simulink model "ES247A_MotAgCmp"  (R2013b)
settings: Solver=VariableStepDiscrete  SolverMode=SingleTasking  StartTime=0.0  StopTime=1  FixedStep=0.002  RelTol=1e-3
values from neighbouring files (symbols this model uses):
  MOTAGCMPENAMASK_CNT_U08 = DataDict.Constant    [ES247A_MotAgCmp_DataDict.m]
  MOTAGCMPMECLDEGPERREV_DEGPERREV_U16P0 = DataDict.Constant    [ES247A_MotAgCmp_DataDict.m]
  MOTAGCUMVALGNDMASK_CNT_U32 = DataDict.Constant    [ES247A_MotAgCmp_DataDict.m]
  MOTAGCUMVALGNDMRFREVMASK_CNT_U32 = DataDict.Constant    [ES247A_MotAgCmp_DataDict.m]
  MOTAGDELTALIM_MOTREV_U0P16 = DataDict.Constant    [ES247A_MotAgCmp_DataDict.m]
  MOTAGMAXDELTA_MOTREV_U0P16 = DataDict.Constant    [ES247A_MotAgCmp_DataDict.m]
  SysGlbPrmMotPoleCnt = DataDict.ImprtdCal    [ES247A_MotAgCmp_DataDict.m]
  SysGlbPrmSysKineRat = DataDict.ImprtdCal    [ES247A_MotAgCmp_DataDict.m]
undefined symbols (not defined in the file or in its folder): sigbuilder_block
libraries: simulink x8, NexteerUtilities x4, FixdToFloat x1
(part 2 of 2)

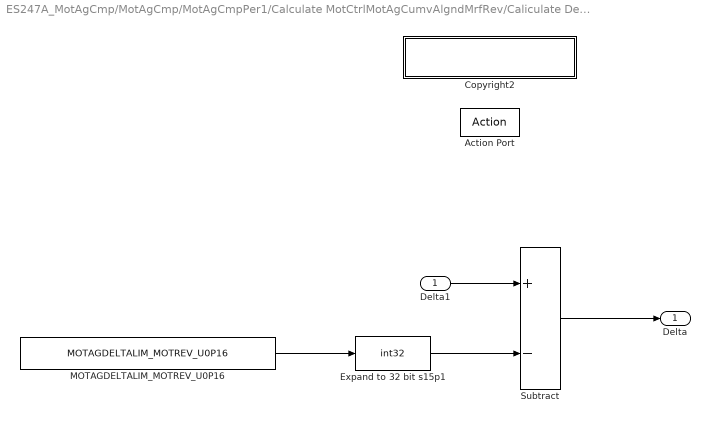
== system ES247A_MotAgCmp/MotAgCmp/MotAgCmpPer1/Calculate MotCtrlMotAgCumvAlgndMrfRev/Caliculate Delta/DeltaCalc/>180 ==
  Delta1 : Inport
  Action Port : ActionPort  ActionType=then
  Copyright2 : Subsystem  Description=|  mask(Copyright Information){none=on}
      | Copyright info block.                                               
      |                                                                     
      | Place copyright information at the top of every subsystem in design.
      mask prompts: none "No parameters"
      mask help: Place copyright information at the top of every subsystem in design.
      mask Display:
      | NxtrConf = 'Nexteer Confidential';
      | 
      | sys = bdroot; %handle for the current model ("system")
      | first = get_param(sys,'Created');
      | if(isempty(first))
      |     first = datestr(now,'yyyy');
      | else
      |     first = first(end-3:end);  %year is last four digits
      | end
      | 
      | last = get_param(sys,'LastModifiedDate');
      | if isempty(last)
      |     last = datestr(now,'yyyy');
      | else
      |     last = last(end-3:end);
      | end
      | 
      | if strcmp(first,last)
      |     fprintf('%s\nCopyright  %s Nexteer',NxtrConf,first);
      | else
      |     fprintf('%s\n%s%s-%s Nexteer',NxtrConf,char(169),first,last);
      | end
  Expand to 32 bit s15p1 : DataTypeConversion  RequirementInfo={} %GIDa_8fa0c183_8262_4d03_9b70_a56e26d42fea  OutDataTypeStr=int32
  MOTAGDELTALIM_MOTREV_U0P16 : Constant  RequirementInfo={} %GIDa_1c78ffbc_90b1_438e_ac1d_71fa1b78e190  Value=MOTAGDELTALIM_MOTREV_U0P16
  Subtract : Sum  Inputs=+-
  Delta : Outport
  wires:
  Delta1/1 -> Subtract/1
  MOTAGDELTALIM_MOTREV_U0P16/1 -> Expand to 32 bit s15p1/1
  Subtract/1 -> Delta/1
  Expand to 32 bit s15p1/1 -> Subtract/2

== system ES247A_MotAgCmp/MotAgCmp/MotAgCmpPer1/Calculate MotCtrlMotAgCumvAlgndMrfRev/Caliculate Delta/DeltaCalc/Copyright2 ==

== system ES247A_MotAgCmp/MotAgCmp/MotAgCmpPer1/Calculate MotCtrlMotAgCumvAlgndMrfRev/Caliculate Delta/DeltaCalc/else ==
  Delta1 : Inport
  Action Port : ActionPort  ActionType=else
  Copyright2 : Subsystem  Description=|  mask(Copyright Information){none=on}
      | Copyright info block.                                               
      |                                                                     
      | Place copyright information at the top of every subsystem in design.
      mask prompts: none "No parameters"
      mask help: Place copyright information at the top of every subsystem in design.
      mask Display:
      | NxtrConf = 'Nexteer Confidential';
      | 
      | sys = bdroot; %handle for the current model ("system")
      | first = get_param(sys,'Created');
      | if(isempty(first))
      |     first = datestr(now,'yyyy');
      | else
      |     first = first(end-3:end);  %year is last four digits
      | end
      | 
      | last = get_param(sys,'LastModifiedDate');
      | if isempty(last)
      |     last = datestr(now,'yyyy');
      | else
      |     last = last(end-3:end);
      | end
      | 
      | if strcmp(first,last)
      |     fprintf('%s\nCopyright  %s Nexteer',NxtrConf,first);
      | else
      |     fprintf('%s\n%s%s-%s Nexteer',NxtrConf,char(169),first,last);
      | end
  Delta : Outport
  wires:
  Delta1/1 -> Delta/1

== system ES247A_MotAgCmp/MotAgCmp/MotAgCmpPer1/Calculate MotCtrlMotAgCumvAlgndMrfRev/Caliculate Delta/DeltaCalc/<(-180)/Copyright2 ==

== system ES247A_MotAgCmp/MotAgCmp/MotAgCmpPer1/Calculate MotCtrlMotAgCumvAlgndMrfRev/Caliculate Delta/DeltaCalc/>180/Copyright2 ==

== system ES247A_MotAgCmp/MotAgCmp/MotAgCmpPer1/Calculate MotCtrlMotAgCumvAlgndMrfRev/Caliculate Delta/DeltaCalc/else/Copyright2 ==

== stateflow chart ES247A_MotAgCmp/MotAgCmp/MotAgCmpPer1/Compute corrected angle and limit to within one electrical rev ==
  (default) -> (junction 2) : {
      | MotCtrlMotAgElec = (SysGlbPrmMotPoleCnt / 2 * MotCtrlMotAgMecl)  - MotAgCmpMotAgBackEmf;
      | }
  (junction 2) -> (junction 6) [order 1] : [
      | MotCtrlMotAgElec < 0
      | ]
      | {
      | MotCtrlMotAgElec = MotCtrlMotAgElec + 65536;
      | }
  (junction 2) -> (junction 9) [order 2] : [
      | MotCtrlMotAgElec >= 65536
      | ]
      | {
      | MotCtrlMotAgElec = MotCtrlMotAgElec - 65536;
      | }
  (junction 9) -> (junction 2)
  (junction 6) -> (junction 2)
  (junction 2) -> (junction 21) [order 3]
  data: MotAgCmpMotAgBackEmf input; MotCtrlMotAgElec output int32; MotCtrlMotAgMecl input; SysGlbPrmMotPoleCnt input

== stateflow chart ES247A_MotAgCmp/SIMULATION ONLY/Function-Call Subsystem/Compute MotAg ==
  (default) -> (junction 2) : {
      | MotAgOut = MotAgIn;
      | }
  (junction 2) -> (junction 6) [order 1] : [
      | MotAgOut < 0
      | ]
      | {
      | MotAgOut = MotAgOut + 65536;
      | }
  (junction 2) -> (junction 9) [order 2] : [
      | MotAgOut >= 65536
      | ]
      | {
      | MotAgOut = MotAgOut - 65536;
      | }
  (junction 9) -> (junction 2)
  (junction 6) -> (junction 2)
  (junction 2) -> (junction 21) [order 3]
  data: MotAgOut output int32; MotAgIn input int32
